simulink model "N3Z_tonetestprevious"  (R2014b)
settings: Solver=ode3  SolverMode=SingleTasking  StartTime=0.0  StopTime=1e-4  FixedStep=fpgaclk  RelTol=1e-3
PreLoadFcn:
  | %fpgaclk=1/32.768e6
  | fpgaclk=1/49.162e6
  | 
  | SerialData=[1,zeros(1,11),1,0,0,1]
  | load ../N3workingG/window
  | win=win';  %Go back to using flatter and wider windowed sync function
  | %load ../N3workingG/hanning    %use Hahn window
  | 
  | load ../N3workingG/PREemphasis   %For pre-empasis and deemphasis FIRs
  | 
  | %LUT3=xls2LUT2('../IQI_Qdemod.xls'); LUT3
  | load ../N3workingG/LUT3
  | load ../N3workingG/FIRiq2
  | % xls2LUT
  | 
  | GetProgFiles
  | 
  | PinAssignments    %Get Pin references for TE0722
  | 
  | 
  | 
  | 
  | 
  | %LCD
  | LCDdata=[LCD_D7,LCD_D6,LCD_D5,LCD_D4,LCD_D3,LCD_D2,LCD_D1,LCD_D0] %Note MSB...LSB!
  | LCDctrl=[LCD_E,LCD_RW,LCD_RS];
  | 
  | %for RS232 on pins 3 and 5 of USBB
  | 
  | %BT chip connections for WT12
  | 
  | RX_BT=RXD
  | TX_BT=TXD
  | 
  | RST_BB=RES
  | 
  | %PCMC=PCMC
  | %PCMS=PCMS
  | %PCMI=PCMI
  | %PCMO=PCMO
  | 
  | %Aliases:
  | SRDBT=PCMI
  | STDBT=PCMO
  | SCLK_BT=PCMC
  | SFS_BT=PCMS
  | 
  | %ADC control
  | 
  | %SDOA=SDOA
  | %SDOB=SDOB
  | %SCK=SCK
  | CONV=Csbar
  | CAL=Cal
  | 
  | ADC_G=[ADC_G3,ADC_G2,ADC_G1,ADC_G0]
  | %PD settings hard coded now
  | 
  | %%%%%%
  | TX_LOW=TX_Low
  | 
  | %Leds
  | %Defined inPinassignments
  | 
  | 
  | 
  | %TouchPads
  | %Defined in Pinassignments
  | load Snip16bSigned
  | 
  | 'Got to end of pre-load OK'
StartFcn:
  | SerialData=[1,zeros(1,11),1,0,0,1]
values from neighbouring files (symbols this model uses):
  ADC_G0 = {'P10'}    [PinAssignments.m]
  ADC_G1 = {'P11'}    [PinAssignments.m]
  ADC_G2 = {'N14'}    [PinAssignments.m]
  ADC_G3 = {'M11'}    [PinAssignments.m]
  Cal = {'L12'}    [PinAssignments.m]
  Csbar = {'M12'}    [PinAssignments.m]
  LCD_D0 = {'J13'}    [PinAssignments.m]
  LCD_D1 = {'J14'}    [PinAssignments.m]
  LCD_D2 = {'F15'}    [PinAssignments.m]
  LCD_D3 = {'H14'}    [PinAssignments.m]
  LCD_D4 = {'G12'}    [PinAssignments.m]
  LCD_D5 = {'L15'}    [PinAssignments.m]
  LCD_D6 = {'M14'}    [PinAssignments.m]
  LCD_D7 = {'K15'}    [PinAssignments.m]
  PCMC = {'H11'}    [PinAssignments.m]
  PCMI = {'H12'}    [PinAssignments.m]
  PCMO = {'N13'}    [PinAssignments.m]
  PCMS = {'M10'}    [PinAssignments.m]
  RES = {'G11'}    [PinAssignments.m]
  RXD = {'H13'}    [PinAssignments.m]
  TX_Low = {'P15'}    [PinAssignments.m]
  TXD = {'P13'}    [PinAssignments.m]
undefined symbols (not defined in the file or in its folder): AXI4, FIRRX, FIRTX, Lite
libraries: xbsIndex_r4 x1250, MyFunctions x43
(part 1 of 10)
settings Model: Creator=Graham  LastModifiedBy=gnaylor
settings DataIOCC: SignalLoggingName=sigsOut
settings OptimizationCC: ExpressionDepthLimit=2147483647  InitFltsAndDblsToZero=on
settings DebuggingCC: SaveWithParameterizedLinksMsg=none  UnderspecifiedInitializationDetection=Classic  MergeDetectMultiDrivingBlocksExec=none  SignalResolutionControl=TryResolveAllWithWarning  SolverPrmCheckMsg=none  MultiTaskDSMMsg=warning  MultiTaskCondExecSysMsg=none  FrameProcessingCompatibilityMsg=error  StateNameClashWarn=warning
settings HardwareCC: TargetUnknown=on
settings GRTTargetCC: TargetFcnLib=ansi_tfl_tmw.mat  ModelReferenceCompliant=off  CombineOutputUpdateFcns=off  MatFileLogging=off  GRTInterface=on

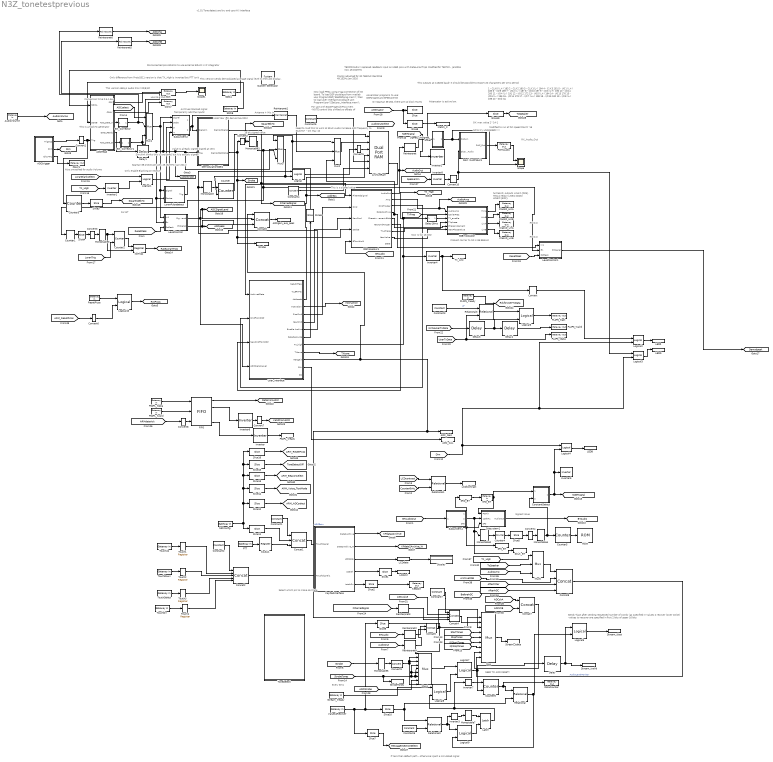
== system N3Z_tonetestprevious ==
  note: If zero then default path - otherwise inject a simulated signal
  note: Every 8ms
  note: Disconnected pico BRAMs to use external BRAM in IP integrator
  note: NEED TO ADD RESET!!
  note: Sends Tlast after sending requested number of words (as specified in Values 2 recover lower 16 bit)
      | -values to recover are specified in first 2 bits of upper 16 bits
  note: Also smoothed for audio Volume
  note: Modified to run at full speed March '16
  note: v1.01 Tone detect and try and use AXI interface
  note: OK max value 2^14-1
  note: This outputs at 115200 baud! It should be possible to export 20 characters per 2ms period
  note: 1 - CLK0 (L+)	183	2 - CLK2	180
      | 3 - CLK1(L-)	184	4 - CLK3	181
      | 5 - I/O1 (L+)	185	6 - I/O9	189
      | 7 - I/O2 (L-)	187	8 - I/O10	197
      | 9 - I/O3 (L+)	190	10 - I/O11	200
      | 11 - I/O4 (L-)	191	12 - I/O12	172
      | 13 - I/O5 (L+)	194	14 - I/O13	176
      | 15 - I/O6 (L-)	196	16 - I/O14	178
      | 17 - I/O7 (L+)	198	18 - I/O15	182
      | 19 - I/O8 (L-)	199	20 - Gnd	NA
  note: This is a 512kHz generator
  note: use 24.6 MHz
  note: Spartan 3E prototype uses 49.152MHz (Jan 2011)
  note: Conversion time 0.5-1.6us
  note: RX_Audio_Out
  note: RF Out
  note: Antenna + Mic In
  note: Now load FPGA using J-tag connection
      | of N3 board.
      | To load DSP picoblaze from matlab use:
      | ProgramDSP('S3eDSPprog.mem');
      | then to load user interface picoblaze use:
      | ProgramUser('S3eUser_interface.mem');
  note: Assembler programs to use:
      | DSPprogN3 and
      | SP3eUserN3
  note: Value is already signed biased at zero
  note: This is a signed value
  note: For use with BootProgMultiPico.mem
      | -NOTE control bits shifted so offsets of
  note: Need to mod this to work at 8kHz Audio
      | Increase ADC frequency to 512kHz? - OK May 10
  note: Closest carrier to N2 is 86.956kHz
  note: 18 bit signed value
  note: Simulink thinks this is unsigned, but it is actualy signed
  note: Clocks adjusted for 32.768MHz Dec2015
      | 49.152Mz Jan 2016
  note: Select which pin to make oscillate
  note: %ClassD_outputs
      | LINA={D25}
      | HINA={B24}
      | LINB={D23}
      | HINB={B22}
  note: RF Out
  note: On Spartan 3E 250, there are 12 block RAMs
  note: NOW try UNSIGNED!!!!!
  note: Temporarily add the inputs!
  note: Now is
      | full 16 bits!
  note: Only difference from Proto2011 version is that TX_High is inverted but PTT isn't
  note: Archives blanked signal
  note: Only enable Blanking on receive
  note: This version delays audio 2ms (20/8/12)
  note: Uses new I_Q demod Nov2012
  note: TEMPORARILY replaced readback input on USER pico with RateLoranTrips
      | Modified for TE0722 - Jan2016 now 49.152MHz
  note: Signed Value
  note: For BT
  note: Attenuator is active low.
  note: This version sends demodulated average signal level to the LCD display.
  " System Generator" : xbsIndex_r4/ System Generator  Tag=genX  xilinxfamily=zynq  part=xc7z010  speed=-1  package=clg225  synthesis_tool=XST  clock_wrapper=Clock Enables  directory=../SysgenOutput/TE0722/ToneDetect2  proj_type=Project Navigator  Synth_file=XST Defaults  Impl_file=ISE Defaults  testbench=off  simulink_period=fpgaclk  sysclk_period=1e9*fpgaclk  dcm_input_clock_period=100  incr_netlist=off  trim_vbits=Everywhere in SubSystem  dbl_ovrd=According to Block Masks  core_generation=According to Block Masks  run_coregen=off  deprecated_control=off  eval_field=0  block_type=sysgen
      settings: block_version=8.2.02
  ADCRead : Subsystem
  ADC_CAL : xbsIndex_r4/Gateway Out  inherit_from_input=off  hdl_port=on  rows=1  columns=1  UseAsDAC=off  DACChannel='1'  interface=None  automatic_assignment=on  address_offset=hex2dec('00')  intf_name=''  intf_description=''  timing_constraint=None  locs_specified=off  LOCs=CAL  io_standard={'LVCMOS33'}  block_type=gatewayout
      settings: block_version=VER_STRING_GOES_HERE
  ADC_Gain : xbsIndex_r4/Gateway Out  inherit_from_input=off  hdl_port=on  rows=1  columns=1  UseAsDAC=off  DACChannel='1'  interface=None  automatic_assignment=on  address_offset=hex2dec('00')  intf_name=''  intf_description=''  timing_constraint=None  locs_specified=on  LOCs=ADC_G  io_standard={'LVCMOS','LVCMOS','LVCMOS','LVCMOS'}  block_type=gatewayout
      settings: block_version=VER_STRING_GOES_HERE
  ADCgain_ave_peak : xbsIndex_r4/Gateway Out  inherit_from_input=off  hdl_port=on  rows=1  columns=1  UseAsDAC=off  DACChannel='1'  interface=AXI4-Lite  automatic_assignment=on  address_offset=hex2dec('00')  intf_name=''  intf_description=''  timing_constraint=None  locs_specified=on  LOCs=Strobe  io_standard={'LVCMOS33'}  block_type=gatewayout
      settings: block_version=VER_STRING_GOES_HERE
  ADCtrigger : Subsystem
  ArchiveRam : xbsIndex_r4/Dual Port RAM  depth=1024*2  initVector=zeros(1,4096)  distributed_mem=Block RAM  init_a=0  init_b=0  rst_a=off  rst_b=off  en_a=off  en_b=off  latency=1  write_mode_A=Read After Write  write_mode_B=Read After Write  optimize=Area  dbl_ovrd=off  block_type=dpram
      settings: block_version=8.2.02
  AudioVolume : xbsIndex_r4/Gateway In  gui_display_data_type=Fixed-point  arith_type=Unsigned  n_bits=9  bin_pt=0  preci_type=Single  exp_width=8  frac_width=24  rows=1  columns=1  quantization="Round  (unbiased: +/- Inf)"  overflow=Saturate  period=fpgaclk  UseAsADC=off  ADCChannel='1'  interface=AXI4-Lite  automatic_assignment=on  address_offset=hex2dec('00')  intf_name=''  intf_description=''  default_value=0  timing_constraint=None  locs_specified=off  LOCs=RS232rx  io_standard={'LVCMOS33'}  inherit_from_input=off  hdl_port=on  dbl_ovrd=off  block_type=gatewayin
      settings: block_version=VER_STRING_GOES_HERE
  Bit_Corrector : Subsystem  TreatAsAtomicUnit=on
  Bit_Corrector1 : Subsystem  TreatAsAtomicUnit=on
  CONV : xbsIndex_r4/Gateway Out  inherit_from_input=off  hdl_port=on  rows=1  columns=1  UseAsDAC=off  DACChannel='1'  interface=None  automatic_assignment=on  address_offset=hex2dec('00')  intf_name=''  intf_description=''  timing_constraint=None  locs_specified=on  LOCs=CONV  io_standard={'LVCMOS33'}  block_type=gatewayout
      settings: xl_area=[0, 0, 0, 0, 0, 0, 0]  block_version=VER_STRING_GOES_HERE
  ClassD_HinA : xbsIndex_r4/Gateway Out  inherit_from_input=off  hdl_port=on  rows=1  columns=1  UseAsDAC=off  DACChannel='1'  interface=None  automatic_assignment=on  address_offset=hex2dec('00')  intf_name=''  intf_description=''  timing_constraint=None  locs_specified=on  LOCs=HINA  io_standard={'LVCMOS33'}  block_type=gatewayout
      settings: xl_area=[0, 0, 0, 0, 0, 0, 0]  block_version=VER_STRING_GOES_HERE
  ClassD_HinB : xbsIndex_r4/Gateway Out  inherit_from_input=off  hdl_port=on  rows=1  columns=1  UseAsDAC=off  DACChannel='1'  interface=None  automatic_assignment=on  address_offset=hex2dec('00')  intf_name=''  intf_description=''  timing_constraint=None  locs_specified=on  LOCs=HINB  io_standard={'LVCMOS33'}  block_type=gatewayout
      settings: xl_area=[0, 0, 0, 0, 0, 0, 0]  block_version=VER_STRING_GOES_HERE
  ClassD_LinA : xbsIndex_r4/Gateway Out  inherit_from_input=off  hdl_port=on  rows=1  columns=1  UseAsDAC=off  DACChannel='1'  interface=None  automatic_assignment=on  address_offset=hex2dec('00')  intf_name=''  intf_description=''  timing_constraint=None  locs_specified=on  LOCs=LINA  io_standard={'LVCMOS33'}  block_type=gatewayout
      settings: xl_area=[0, 0, 0, 0, 0, 0, 0]  block_version=VER_STRING_GOES_HERE
  ClassD_LinB : xbsIndex_r4/Gateway Out  inherit_from_input=off  hdl_port=on  rows=1  columns=1  UseAsDAC=off  DACChannel='1'  interface=None  automatic_assignment=on  address_offset=hex2dec('00')  intf_name=''  intf_description=''  timing_constraint=None  locs_specified=on  LOCs=LINB  io_standard={'LVCMOS33'}  block_type=gatewayout
      settings: xl_area=[0, 0, 0, 0, 0, 0, 0]  block_version=VER_STRING_GOES_HERE
  Concat1 : xbsIndex_r4/Concat  num_inputs=3  dbl_ovrd=off  block_type=concat
      settings: block_version=12.2
  Concat2 : xbsIndex_r4/Concat  num_inputs=5  dbl_ovrd=off  block_type=concat
      settings: block_version=12.2
  Concat4 : xbsIndex_r4/Concat  num_inputs=4  dbl_ovrd=off  block_type=concat
  Concat5 : xbsIndex_r4/Concat  num_inputs=2  dbl_ovrd=off  block_type=concat
  Concat6 : xbsIndex_r4/Concat  num_inputs=3  dbl_ovrd=off  block_type=concat
  Concat7 : xbsIndex_r4/Concat  num_inputs=2  dbl_ovrd=off  block_type=concat
  Concat8 : xbsIndex_r4/Concat  num_inputs=4  dbl_ovrd=off  block_type=concat
  Constant1 : xbsIndex_r4/Constant  const=0  gui_display_data_type=Fixed-point  arith_type=Unsigned  n_bits=4  bin_pt=0  preci_type=Single  exp_width=8  frac_width=24  explicit_period=on  period=fpgaclk  equ=P=C  opselect=C  inp2=PCIN>>17  opr=+  inp1=P  carry=CIN  dbl_ovrd=off  block_type=constant
      settings: block_version=VER_STRING_GOES_HERE
  Constant2 : xbsIndex_r4/Constant  const=0  gui_display_data_type=Fixed-point  arith_type=Unsigned  n_bits=4  bin_pt=0  preci_type=Single  exp_width=8  frac_width=24  explicit_period=on  period=fpgaclk  equ=P=C  opselect=C  inp2=PCIN>>17  opr=+  inp1=P  carry=CIN  dbl_ovrd=off  block_type=constant
      settings: block_version=VER_STRING_GOES_HERE
  Constant3 : xbsIndex_r4/Constant  const=10  gui_display_data_type=Fixed-point  arith_type=Unsigned  n_bits=8  bin_pt=0  preci_type=Single  exp_width=8  frac_width=24  explicit_period=off  period=1  equ=P=C  opselect=C  inp2=PCIN>>17  opr=+  inp1=P  carry=CIN  dbl_ovrd=off  block_type=constant
  Constant4 : xbsIndex_r4/Constant  const=0  gui_display_data_type=Boolean  arith_type=Boolean  n_bits=1  bin_pt=0  preci_type=Single  exp_width=8  frac_width=24  explicit_period=on  period=fpgaclk  equ=P=C  opselect=C  inp2=PCIN>>17  opr=+  inp1=P  carry=CIN  dbl_ovrd=off  block_type=constant
      settings: block_version=VER_STRING_GOES_HERE
  Constant5 : xbsIndex_r4/Constant  const=0  gui_display_data_type=Fixed-point  arith_type=Unsigned  n_bits=16  bin_pt=0  preci_type=Single  exp_width=8  frac_width=24  explicit_period=on  period=fpgaclk  equ=P=C  opselect=C  inp2=PCIN>>17  opr=+  inp1=P  carry=CIN  dbl_ovrd=off  block_type=constant
      settings: block_version=VER_STRING_GOES_HERE
  Constant6 : xbsIndex_r4/Constant  const=0  gui_display_data_type=Fixed-point  arith_type=Unsigned  n_bits=16  bin_pt=0  preci_type=Single  exp_width=8  frac_width=24  explicit_period=on  period=fpgaclk  equ=P=C  opselect=C  inp2=PCIN>>17  opr=+  inp1=P  carry=CIN  dbl_ovrd=off  block_type=constant
  Constant7 : xbsIndex_r4/Constant  const=0  gui_display_data_type=Fixed-point  arith_type=Unsigned  n_bits=2  bin_pt=0  preci_type=Single  exp_width=8  frac_width=24  explicit_period=on  period=fpgaclk  equ=P=C  opselect=C  inp2=PCIN>>17  opr=+  inp1=P  carry=CIN  dbl_ovrd=off  block_type=constant
  ConstantDetect : Subsystem
  Convert : xbsIndex_r4/Convert  gui_display_data_type=Boolean  arith_type=Boolean  n_bits=16  bin_pt=14  float_type=Single  exp_bits=8  fraction_bits=24  quantization=Truncate  overflow=Wrap  en=off  latency=0  pipeline=off  dbl_ovrd=off  block_type=convert
      settings: block_version=8.2.02
  Convert1 : xbsIndex_r4/Convert  gui_display_data_type=Boolean  arith_type=Boolean  n_bits=8  bin_pt=6  float_type=Single  exp_bits=8  fraction_bits=24  quantization=Truncate  overflow=Wrap  en=off  latency=0  pipeline=off  dbl_ovrd=off  block_type=convert
      settings: xl_area=[0 0 0 0 0 0 0]  block_version=VER_STRING_GOES_HERE
  Convert10 : xbsIndex_r4/Convert  gui_display_data_type=Boolean  arith_type=Boolean  n_bits=16  bin_pt=14  float_type=Single  exp_bits=8  fraction_bits=24  quantization=Truncate  overflow=Wrap  en=off  latency=0  pipeline=off  dbl_ovrd=off  block_type=convert
      settings: block_version=8.2.02
  Convert2 : xbsIndex_r4/Convert  gui_display_data_type=Boolean  arith_type=Boolean  n_bits=16  bin_pt=0  float_type=Single  exp_bits=8  fraction_bits=24  quantization=Truncate  overflow=Wrap  en=off  latency=0  pipeline=off  dbl_ovrd=off  block_type=convert
      settings: xl_area=[0, 0, 0, 0, 0, 0, 0]  block_version=VER_STRING_GOES_HERE
  Convert3 : xbsIndex_r4/Convert  gui_display_data_type=Fixed-point  arith_type=Boolean  n_bits=16  bin_pt=14  float_type=Single  exp_bits=8  fraction_bits=24  quantization=Truncate  overflow=Wrap  en=off  latency=0  pipeline=off  dbl_ovrd=off  block_type=convert
      settings: block_version=8.2.02
  Convert4 : xbsIndex_r4/Convert  gui_display_data_type=Fixed-point  arith_type=Boolean  n_bits=8  bin_pt=6  float_type=Single  exp_bits=8  fraction_bits=24  quantization=Truncate  overflow=Wrap  en=off  latency=0  pipeline=off  dbl_ovrd=off  block_type=convert
      settings: xl_area=[0 0 0 0 0 0 0]  block_version=VER_STRING_GOES_HERE
  Convert5 : xbsIndex_r4/Convert  gui_display_data_type=Fixed-point  arith_type=Boolean  n_bits=16  bin_pt=14  float_type=Single  exp_bits=8  fraction_bits=24  quantization=Truncate  overflow=Wrap  en=off  latency=0  pipeline=off  dbl_ovrd=off  block_type=convert
      settings: block_version=8.2.02
  Convert6 : xbsIndex_r4/Convert  gui_display_data_type=Boolean  arith_type=Boolean  n_bits=8  bin_pt=6  float_type=Single  exp_bits=8  fraction_bits=24  quantization=Truncate  overflow=Wrap  en=off  latency=0  pipeline=off  dbl_ovrd=off  block_type=convert
      settings: xl_area=[0 0 0 0 0 0 0]  block_version=VER_STRING_GOES_HERE
  Convert7 : xbsIndex_r4/Convert  gui_display_data_type=Fixed-point  arith_type=Unsigned  n_bits=1  bin_pt=0  float_type=Single  exp_bits=8  fraction_bits=24  quantization=Truncate  overflow=Wrap  en=off  latency=0  pipeline=off  dbl_ovrd=off  block_type=convert
      settings: block_version=8.2.02
  Convert8 : xbsIndex_r4/Convert  gui_display_data_type=Boolean  arith_type=Boolean  n_bits=1  bin_pt=0  float_type=Single  exp_bits=8  fraction_bits=24  quantization=Truncate  overflow=Wrap  en=off  latency=0  pipeline=off  dbl_ovrd=off  block_type=convert
      settings: block_version=8.2.02
  Convert9 : xbsIndex_r4/Convert  gui_display_data_type=Boolean  arith_type=Boolean  n_bits=16  bin_pt=14  float_type=Single  exp_bits=8  fraction_bits=24  quantization=Truncate  overflow=Wrap  en=off  latency=1  pipeline=off  dbl_ovrd=off  block_type=convert
  Counter : xbsIndex_r4/Counter  cnt_type=Free Running  cnt_to=Inf  operation=Up  start_count=0  cnt_by_val=1  arith_type=Unsigned  n_bits=11  bin_pt=0  load_pin=off  rst=on  en=on  explicit_period=off  period=1  use_behavioral_HDL=off  implementation=Fabric  use_rpm=off  dbl_ovrd=off  block_type=counter
      settings: block_version=8.2.02
  Counter1 : xbsIndex_r4/Counter  cnt_type=Free Running  cnt_to=Inf  operation=Up  start_count=0  cnt_by_val=1  arith_type=Unsigned  n_bits=13  bin_pt=0  load_pin=off  rst=off  en=on  explicit_period=off  period=1  use_behavioral_HDL=off  implementation=Fabric  use_rpm=off  dbl_ovrd=off  block_type=counter
      settings: block_version=8.2.02
  Counter2 : xbsIndex_r4/Counter  cnt_type=Free Running  cnt_to=Inf  operation=Up  start_count=0  cnt_by_val=1  arith_type=Unsigned  n_bits=8  bin_pt=0  load_pin=off  rst=on  en=on  explicit_period=off  period=1  use_behavioral_HDL=off  implementation=Fabric  use_rpm=off  dbl_ovrd=off  block_type=counter
      settings: block_version=8.2.02
  Counter3 : xbsIndex_r4/Counter  cnt_type=Free Running  cnt_to=Inf  operation=Up  start_count=0  cnt_by_val=1  arith_type=Unsigned  n_bits=2  bin_pt=0  load_pin=off  rst=off  en=on  explicit_period=on  period=fpgaclk  use_behavioral_HDL=off  implementation=Fabric  dbl_ovrd=off  block_type=counter
      settings: block_version=12.2
  Counter4 : xbsIndex_r4/Counter  cnt_type=Free Running  cnt_to=Inf  operation=Up  start_count=0  cnt_by_val=1  arith_type=Unsigned  n_bits=4  bin_pt=0  load_pin=off  rst=off  en=on  explicit_period=on  period=fpgaclk  use_behavioral_HDL=off  implementation=Fabric  dbl_ovrd=off  block_type=counter
      settings: block_version=12.2
  Counter5 : xbsIndex_r4/Counter  cnt_type=Free Running  cnt_to=Inf  operation=Up  start_count=0  cnt_by_val=1  arith_type=Unsigned  n_bits=4  bin_pt=0  load_pin=off  rst=off  en=on  explicit_period=on  period=fpgaclk  use_behavioral_HDL=off  implementation=Fabric  dbl_ovrd=off  block_type=counter
  Counter6 : xbsIndex_r4/Counter  cnt_type=Free Running  cnt_to=Inf  operation=Up  start_count=0  cnt_by_val=1  arith_type=Unsigned  n_bits=16  bin_pt=0  load_pin=off  rst=on  en=on  explicit_period=on  period=fpgaclk  use_behavioral_HDL=off  implementation=Fabric  dbl_ovrd=off  block_type=counter
  CoutA1 : xbsIndex_r4/Register  init=0  rst=off  en=off  dbl_ovrd=off  block_type=register
      settings: xl_area=[0, 0, 0, 0, 0, 0, 0]  block_version=VER_STRING_GOES_HERE
  DAC (XAPP154)1 : Subsystem
  DSProcessor1 : Subsystem
  DataCounter : xbsIndex_r4/Gateway Out  inherit_from_input=off  hdl_port=on  rows=1  columns=1  UseAsDAC=off  DACChannel='1'  interface=None  automatic_assignment=on  address_offset=hex2dec('00')  intf_name=''  intf_description=''  timing_constraint=None  locs_specified=off  LOCs=Keep_On  io_standard={'LVCMOS33'}  block_type=gatewayout
      settings: xl_area=[0, 0, 0, 0, 0, 0, 0]  block_version=VER_STRING_GOES_HERE
  Delay : xbsIndex_r4/Delay  rst=off  infoeditControl=Selection of Reset will increase slice count due to use of real FFs and instead of SRLs  en=off  latency=2  reg_retiming=off  dbl_ovrd=off  block_type=delay
      settings: infoedit=Hardware notes: A delay line is a chain, each link of which is an SRL16 or SRL32 followed by a flip-flop.
  Delay1 : xbsIndex_r4/Delay  rst=off  infoeditControl=Selection of Reset will increase slice count due to use of real FFs and instead of SRLs  en=off  latency=2  reg_retiming=off  dbl_ovrd=off  block_type=delay
      settings: xl_area=[1 1 0 0 0 0 0]  block_version=VER_STRING_GOES_HERE
  Delay16ms : Subsystem
  Delay3 : xbsIndex_r4/Delay  rst=off  infoeditControl=Selection of Reset will increase slice count due to use of real FFs and instead of SRLs  en=off  latency=2  reg_retiming=off  dbl_ovrd=off  block_type=delay
      settings: infoedit=Hardware notes: A delay line is a chain, each link of which is an SRL16 or SRL32 followed by a flip-flop.
  Delay4 : xbsIndex_r4/Delay  rst=off  infoeditControl=Selection of Reset will increase slice count due to use of real FFs and instead of SRLs  en=off  latency=1  reg_retiming=off  dbl_ovrd=off  block_type=delay
      settings: infoedit=Hardware notes: A delay line is a chain, each link of which is an SRL16 or SRL32 followed by a flip-flop.
  DemodulationSSB1 : Subsystem
  Display : Display
  FIFO : xbsIndex_r4/FIFO  mem_type=Block RAM  performance_options=First_Word_Fall_Through  embedded_registers=on  depth=16  percent_nbits=1  rst=off  rst_latency=1  en=off  use_dcount=off  use_percent_full_port=off  use_almost_empty=off  almost_empty_thresh=2  use_almost_full=on  almost_full_thresh=14  explicit_period=off  dbl_ovrd=off  block_type=fifo
  Inverter{,1..2,4..6,8} (7 alike) : xbsIndex_r4/Inverter  en=off  latency=0  dbl_ovrd=off  block_type=inv
      Inverter1 settings: block_version=12.2
      Inverter2 settings: block_version=12.2
      Inverter4 settings: block_version=12.2
      Inverter5 settings: block_version=12.2
      Inverter8 settings: block_version=12.2
  Inverter3 : xbsIndex_r4/Inverter  en=off  latency=1  dbl_ovrd=off  block_type=inv
  Inverter7 : xbsIndex_r4/Inverter  en=off  latency=1  dbl_ovrd=off  block_type=inv
  KeepOn : xbsIndex_r4/Gateway Out  inherit_from_input=off  hdl_port=on  rows=1  columns=1  UseAsDAC=off  DACChannel='1'  interface=None  automatic_assignment=on  address_offset=hex2dec('00')  intf_name=''  intf_description=''  timing_constraint=None  locs_specified=on  LOCs=Keep_On  io_standard={'LVCMOS33'}  block_type=gatewayout
      settings: xl_area=[0, 0, 0, 0, 0, 0, 0]  block_version=VER_STRING_GOES_HERE
  KeyPadinterface : Subsystem
  LCDContrast : xbsIndex_r4/Gateway Out  inherit_from_input=off  hdl_port=on  rows=1  columns=1  UseAsDAC=off  DACChannel='1'  interface=None  automatic_assignment=on  address_offset=hex2dec('00')  intf_name=''  intf_description=''  timing_constraint=None  locs_specified=on  LOCs=LCD_V0  io_standard={'LVCMOS33'}  block_type=gatewayout
      settings: block_version=VER_STRING_GOES_HERE
  LCDctrl : xbsIndex_r4/Gateway Out  inherit_from_input=off  hdl_port=on  rows=1  columns=1  UseAsDAC=off  DACChannel='1'  interface=None  automatic_assignment=on  address_offset=hex2dec('00')  intf_name=''  intf_description=''  timing_constraint=None  locs_specified=on  LOCs=LCDctrl  io_standard={'LVCMOS33','LVCMOS33','LVCMOS33'}  block_type=gatewayout
      settings: block_version=VER_STRING_GOES_HERE
  LCDdata : xbsIndex_r4/Gateway Out  inherit_from_input=off  hdl_port=on  rows=1  columns=1  UseAsDAC=off  DACChannel='1'  interface=None  automatic_assignment=on  address_offset=hex2dec('00')  intf_name=''  intf_description=''  timing_constraint=None  locs_specified=on  LOCs=LCDdata  io_standard={'LVCMOS33','LVCMOS33','LVCMOS33','LVCMOS33','LVCMOS33','LVCMOS33','LVCMOS33','LVCMOS33'}  block_type=gatewayout
      settings: block_version=VER_STRING_GOES_HERE
  LEDB : xbsIndex_r4/Gateway Out  inherit_from_input=off  hdl_port=on  rows=1  columns=1  UseAsDAC=off  DACChannel='1'  interface=None  automatic_assignment=on  address_offset=hex2dec('00')  intf_name=''  intf_description=''  timing_constraint=None  locs_specified=on  LOCs=RGB_B  io_standard={'LVCMOS33'}  block_type=gatewayout
      settings: block_version=VER_STRING_GOES_HERE
  LEDG : xbsIndex_r4/Gateway Out  inherit_from_input=off  hdl_port=on  rows=1  columns=1  UseAsDAC=off  DACChannel='1'  interface=None  automatic_assignment=on  address_offset=hex2dec('00')  intf_name=''  intf_description=''  timing_constraint=None  locs_specified=on  LOCs=RGB_G  io_standard={'LVCMOS33'}  block_type=gatewayout
      settings: block_version=VER_STRING_GOES_HERE
  LEDR : xbsIndex_r4/Gateway Out  inherit_from_input=off  hdl_port=on  rows=1  columns=1  UseAsDAC=off  DACChannel='1'  interface=None  automatic_assignment=on  address_offset=hex2dec('00')  intf_name=''  intf_description=''  timing_constraint=None  locs_specified=on  LOCs=RGB_R  io_standard={'LVCMOS33'}  block_type=gatewayout
      settings: block_version=VER_STRING_GOES_HERE
  Latch : MyFunctions/Latch
  LevelMonitor : Subsystem
  LevelMonitor1 : Subsystem
  Logical : xbsIndex_r4/Logical  logical_function=AND  inputs=2  en=off  latency=2  precision=Full  arith_type=Unsigned  n_bits=16  bin_pt=0  align_bp=on  dbl_ovrd=off  block_type=logical
      settings: block_version=8.2.02
  Logical1 : xbsIndex_r4/Logical  logical_function=AND  inputs=2  en=off  latency=1  precision=Full  arith_type=Unsigned  n_bits=16  bin_pt=0  align_bp=on  dbl_ovrd=off  block_type=logical
      settings: block_version=8.2.02
  Logical{2..4,10} (4 alike) : xbsIndex_r4/Logical  logical_function=OR  inputs=2  en=off  latency=1  precision=Full  arith_type=Unsigned  n_bits=16  bin_pt=0  align_bp=on  dbl_ovrd=off  block_type=logical
  Logical5 : xbsIndex_r4/Logical  logical_function=AND  inputs=2  en=off  latency=0  precision=Full  arith_type=Unsigned  n_bits=16  bin_pt=0  align_bp=on  dbl_ovrd=off  block_type=logical
  Logical6 : xbsIndex_r4/Logical  logical_function=AND  inputs=2  en=off  latency=1  precision=Full  arith_type=Unsigned  n_bits=16  bin_pt=0  align_bp=on  dbl_ovrd=off  block_type=logical
  Logical7 : xbsIndex_r4/Logical  logical_function=AND  inputs=2  en=off  latency=1  precision=Full  arith_type=Unsigned  n_bits=16  bin_pt=0  align_bp=on  dbl_ovrd=off  block_type=logical
  Logical8 : xbsIndex_r4/Logical  logical_function=AND  inputs=2  en=off  latency=0  precision=Full  arith_type=Unsigned  n_bits=16  bin_pt=0  align_bp=on  dbl_ovrd=off  block_type=logical
  Logical9 : xbsIndex_r4/Logical  logical_function=OR  inputs=2  en=off  latency=0  precision=Full  arith_type=Unsigned  n_bits=16  bin_pt=0  align_bp=on  dbl_ovrd=off  block_type=logical
  LoranPulsedetect : Subsystem
  Match_Z : xbsIndex_r4/Gateway Out  inherit_from_input=off  hdl_port=on  rows=1  columns=1  UseAsDAC=off  DACChannel='1'  interface=None  automatic_assignment=on  address_offset=hex2dec('00')  intf_name=''  intf_description=''  timing_constraint=None  locs_specified=on  LOCs=MatchZ  io_standard={'LVCMOS33'}  block_type=gatewayout
      settings: block_version=VER_STRING_GOES_HERE
  Monostable : MyFunctions/Monostable
  Monostable1 : MyFunctions/Monostable
      link override Delay1: en=off  latency=1  dbl_ovrd=off  reg_retiming=off
      link override Delay1: infoedit=Hardware notes: A delay line is a chain, each link of which is an SRL16 followed by a flip-flop.  xl_area=[0, 0, 0, 0, 0, 0, 0]
  Monostable2 : MyFunctions/Monostable
      link override Delay1: xl_area=[1 1 0 0 0 0 0]
      link override Inverter: xl_area=[0 0 0 0 0 0 0]
      link override Logical: xl_area=[1 0 0 1 0 0 0]
  Monostable3 : MyFunctions/Monostable
      link override Delay1: en=off  latency=1  dbl_ovrd=off  reg_retiming=off
      link override Delay1: infoedit=Hardware notes: A delay line is a chain, each link of which is an SRL16 followed by a flip-flop.  xl_area=[0, 0, 0, 0, 0, 0, 0]
  Monostable4 : MyFunctions/Monostable
      link override Delay1: xl_area=[1 1 0 0 0 0 0]
      link override Inverter: xl_area=[0 0 0 0 0 0 0]
      link override Logical: xl_area=[1 0 0 1 0 0 0]
  Monostable5 : MyFunctions/Monostable
      link override Delay1: en=off  latency=1  dbl_ovrd=off  reg_retiming=off
      link override Delay1: infoedit=Hardware notes: A delay line is a chain, each link of which is an SRL16 followed by a flip-flop.  xl_area=[0, 0, 0, 0, 0, 0, 0]
  Monostable7 : MyFunctions/Monostable
      link override Delay1: en=off  latency=1  dbl_ovrd=off  reg_retiming=off
      link override Delay1: infoedit=Hardware notes: A delay line is a chain, each link of which is an SRL16 followed by a flip-flop.  xl_area=[0, 0, 0, 0, 0, 0, 0]
  Mux : xbsIndex_r4/Mux  inputs=8  en=off  latency=1  precision=Full  arith_type=Unsigned  n_bits=16  bin_pt=14  quantization=Truncate  overflow=Wrap  dbl_ovrd=off  block_type=mux
  Mux{1..3,5} (4 alike) : xbsIndex_r4/Mux  inputs=2  en=off  latency=1  precision=Full  arith_type=Unsigned  n_bits=16  bin_pt=14  quantization=Truncate  overflow=Wrap  dbl_ovrd=off  block_type=mux
      Mux1 settings: block_version=VER_STRING_GOES_HERE
      Mux2 settings: block_version=VER_STRING_GOES_HERE
      Mux3 settings: block_version=VER_STRING_GOES_HERE
  Mux4 : xbsIndex_r4/Mux  inputs=8  en=off  latency=1  precision=Full  arith_type=Unsigned  n_bits=16  bin_pt=14  quantization=Truncate  overflow=Wrap  dbl_ovrd=off  block_type=mux
  N3Zconfig : xbsIndex_r4/Gateway In  gui_display_data_type=Fixed-point  arith_type=Unsigned  n_bits=32  bin_pt=0  preci_type=Single  exp_width=8  frac_width=24  rows=1  columns=1  quantization=Truncate  overflow=Saturate  period=fpgaclk  UseAsADC=off  ADCChannel='1'  interface=AXI4-Lite  automatic_assignment=on  address_offset=hex2dec('00')  intf_name=''  intf_description=''  default_value=0  timing_constraint=None  locs_specified=off  LOCs=PTT  io_standard={'LVCMOS33'}  inherit_from_input=off  hdl_port=on  dbl_ovrd=off  block_type=gatewayin
      settings: xl_area=[0, 0, 0, 0, 0, 0, 0]  block_version=VER_STRING_GOES_HERE
  NoTrips : xbsIndex_r4/Register  init=0  rst=off  en=on  dbl_ovrd=off  block_type=register
      settings: xl_area=[0, 0, 0, 0, 0, 0, 0]  block_version=VER_STRING_GOES_HERE
  PL2PS_tdata : xbsIndex_r4/Gateway Out  inherit_from_input=off  hdl_port=on  rows=1  columns=1  UseAsDAC=off  DACChannel='1'  interface=None  automatic_assignment=on  address_offset=hex2dec('00')  intf_name=''  intf_description=''  timing_constraint=None  locs_specified=off  LOCs={}  io_standard={}  block_type=gatewayout
  PL2PS_tlast : xbsIndex_r4/Gateway Out  inherit_from_input=off  hdl_port=on  rows=1  columns=1  UseAsDAC=off  DACChannel='1'  interface=None  automatic_assignment=on  address_offset=hex2dec('00')  intf_name=''  intf_description=''  timing_constraint=None  locs_specified=off  LOCs={}  io_standard={}  block_type=gatewayout
  PL2PS_tready : xbsIndex_r4/Gateway In  gui_display_data_type=Boolean  arith_type=Boolean  n_bits=1  bin_pt=0  preci_type=Single  exp_width=8  frac_width=24  rows=1  columns=1  quantization="Round  (unbiased: +/- Inf)"  overflow=Wrap  period=fpgaclk  UseAsADC=off  ADCChannel='1'  interface=None  automatic_assignment=on  address_offset=hex2dec('00')  intf_name=''  intf_description=''  default_value=0  timing_constraint=None  locs_specified=off  LOCs=RS232rx  io_standard={'LVCMOS33'}  inherit_from_input=off  hdl_port=on  dbl_ovrd=off  block_type=gatewayin
      settings: block_version=VER_STRING_GOES_HERE
  PL2PS_tvalid : xbsIndex_r4/Gateway Out  inherit_from_input=off  hdl_port=on  rows=1  columns=1  UseAsDAC=off  DACChannel='1'  interface=None  automatic_assignment=on  address_offset=hex2dec('00')  intf_name=''  intf_description=''  timing_constraint=None  locs_specified=off  LOCs={}  io_standard={}  block_type=gatewayout
  PS2PL_tdata : xbsIndex_r4/Gateway In  gui_display_data_type=Fixed-point  arith_type=Unsigned  n_bits=8  bin_pt=0  preci_type=Single  exp_width=8  frac_width=24  rows=1  columns=1  quantization="Round  (unbiased: +/- Inf)"  overflow=Wrap  period=fpgaclk  UseAsADC=off  ADCChannel='1'  interface=None  automatic_assignment=on  address_offset=hex2dec('00')  intf_name=''  intf_description=''  default_value=0  timing_constraint=None  locs_specified=off  LOCs=RS232rx  io_standard={'LVCMOS33'}  inherit_from_input=off  hdl_port=on  dbl_ovrd=off  block_type=gatewayin
      settings: block_version=VER_STRING_GOES_HERE
  PS2PL_tready : xbsIndex_r4/Gateway Out  inherit_from_input=off  hdl_port=on  rows=1  columns=1  UseAsDAC=off  DACChannel='1'  interface=None  automatic_assignment=on  address_offset=hex2dec('00')  intf_name=''  intf_description=''  timing_constraint=None  locs_specified=off  LOCs=RST_BB  io_standard={'LVCMOS'}  block_type=gatewayout
      settings: block_version=VER_STRING_GOES_HERE
  PS2PL_tvalid : xbsIndex_r4/Gateway In  gui_display_data_type=Boolean  arith_type=Boolean  n_bits=1  bin_pt=0  preci_type=Single  exp_width=8  frac_width=24  rows=1  columns=1  quantization="Round  (unbiased: +/- Inf)"  overflow=Wrap  period=fpgaclk  UseAsADC=off  ADCChannel='1'  interface=None  automatic_assignment=on  address_offset=hex2dec('00')  intf_name=''  intf_description=''  default_value=0  timing_constraint=None  locs_specified=off  LOCs=RS232rx  io_standard={'LVCMOS33'}  inherit_from_input=off  hdl_port=on  dbl_ovrd=off  block_type=gatewayin
      settings: block_version=VER_STRING_GOES_HERE
  PSUclk : xbsIndex_r4/Gateway Out  inherit_from_input=off  hdl_port=on  rows=1  columns=1  UseAsDAC=off  DACChannel='1'  interface=None  automatic_assignment=on  address_offset=hex2dec('00')  intf_name=''  intf_description=''  timing_constraint=None  locs_specified=off  LOCs={}  io_standard={}  block_type=gatewayout
  PTT : xbsIndex_r4/Gateway In  gui_display_data_type=Fixed-point  arith_type=Unsigned  n_bits=1  bin_pt=0  preci_type=Single  exp_width=8  frac_width=24  rows=1  columns=1  quantization=Truncate  overflow=Saturate  period=fpgaclk  UseAsADC=off  ADCChannel='1'  interface=None  automatic_assignment=on  address_offset=hex2dec('00')  intf_name=''  intf_description=''  default_value=0  timing_constraint=None  locs_specified=on  LOCs=PTT  io_standard={'LVCMOS33'}  inherit_from_input=off  hdl_port=on  dbl_ovrd=off  block_type=gatewayin
      settings: xl_area=[0, 0, 0, 0, 0, 0, 0]  block_version=VER_STRING_GOES_HERE
  PWMAudio : xbsIndex_r4/Gateway Out  inherit_from_input=off  hdl_port=on  rows=1  columns=1  UseAsDAC=off  DACChannel='1'  interface=None  automatic_assignment=on  address_offset=hex2dec('00')  intf_name=''  intf_description=''  timing_constraint=None  locs_specified=on  LOCs=PWMAudio  io_standard={'LVCMOS33'}  block_type=gatewayout
      settings: xl_area=[0, 0, 0, 0, 0, 0, 0]  block_version=VER_STRING_GOES_HERE
  ROM : xbsIndex_r4/ROM  depth=16  initVector=(2^14-2^12)*sin(pi*(0:15)/8)  distributed_mem=Distributed memory  rst=off  init_reg=0  en=off  latency=1  gui_display_data_type=Fixed-point  arith_type="Signed  (2's comp)"  n_bits=16  bin_pt=0  preci_type=Single  exp_width=8  frac_width=24  optimize=Area  use_rpm=on  dbl_ovrd=off  block_type=sprom
  Reinterpret : xbsIndex_r4/Reinterpret  force_arith_type=on  arith_type="Signed  (2's comp)"  force_bin_pt=on  bin_pt=0  block_type=cast
      settings: block_version=VER_STRING_GOES_HERE
  Reinterpret1 : xbsIndex_r4/Reinterpret  force_arith_type=on  arith_type=Unsigned  force_bin_pt=on  bin_pt=0  block_type=reinterpret
      settings: infoedit="Changes signal type without altering the binary representation.   You can changed the signal between signed and unsigned, and relocate the binary point.<br><br>Hardware notes: In hardware this block costs nothing.<br><br>Example:  Suppose the input is 6 bits wide, signed, with 2 fractional bits, and the output is forced to unsigned with 0 fractional bits.  Then an input of -2.0 (1110.00 in binary 2's complement) becomes an output of 56 (111000 in binary)."  block_version=8.2.02
  Reinterpret2 : xbsIndex_r4/Reinterpret  force_arith_type=on  arith_type=Unsigned  force_bin_pt=on  bin_pt=0  block_type=cast
      settings: block_version=VER_STRING_GOES_HERE
  Reinterpret3 : xbsIndex_r4/Reinterpret  force_arith_type=on  arith_type=Unsigned  force_bin_pt=on  bin_pt=0  block_type=cast
      settings: block_version=VER_STRING_GOES_HERE
  Reinterpret4 : xbsIndex_r4/Reinterpret  force_arith_type=on  arith_type=Unsigned  force_bin_pt=on  bin_pt=0  block_type=cast
      settings: block_version=VER_STRING_GOES_HERE
  Reinterpret5 : xbsIndex_r4/Reinterpret  force_arith_type=on  arith_type=Unsigned  force_bin_pt=on  bin_pt=0  block_type=reinterpret
      settings: block_version=8.2.02
  Reinterpret6 : xbsIndex_r4/Reinterpret  force_arith_type=on  arith_type=Unsigned  force_bin_pt=on  bin_pt=0  block_type=reinterpret
      settings: block_version=8.2.02
  Relational : xbsIndex_r4/Relational  mode=a=b  op_type=Bool  en=off  latency=1  dbl_ovrd=off  block_type=relational
  Relational1 : xbsIndex_r4/Relational  mode=a>b  op_type=Bool  en=off  latency=1  dbl_ovrd=off  block_type=relational
      settings: block_version=10.1
  Relational2 : xbsIndex_r4/Relational  mode=a=b  op_type=Bool  en=off  latency=1  dbl_ovrd=off  block_type=relational
  Relational3 : xbsIndex_r4/Relational  mode=a=b  op_type=Bool  en=off  latency=1  dbl_ovrd=off  block_type=relational
  ResetPicos : xbsIndex_r4/Gateway In  gui_display_data_type=Boolean  arith_type=Boolean  n_bits=1  bin_pt=0  preci_type=Single  exp_width=8  frac_width=24  rows=1  columns=1  quantization="Round  (unbiased: +/- Inf)"  overflow=Saturate  period=fpgaclk  UseAsADC=off  ADCChannel='1'  interface=None  automatic_assignment=on  address_offset=hex2dec('00')  intf_name=''  intf_description=''  default_value=0  timing_constraint=None  locs_specified=off  LOCs=RS232rx  io_standard={'LVCMOS33'}  inherit_from_input=off  hdl_port=on  dbl_ovrd=off  block_type=gatewayin
      settings: block_version=VER_STRING_GOES_HERE
  SCK : xbsIndex_r4/Gateway Out  inherit_from_input=off  hdl_port=on  rows=1  columns=1  UseAsDAC=off  DACChannel='1'  interface=None  automatic_assignment=on  address_offset=hex2dec('00')  intf_name=''  intf_description=''  timing_constraint=None  locs_specified=on  LOCs=SCK  io_standard={'LVCMOS33'}  block_type=gatewayout
      settings: xl_area=[0, 0, 0, 0, 0, 0, 0]  block_version=VER_STRING_GOES_HERE
  SCLK_BT : xbsIndex_r4/Gateway Out  inherit_from_input=off  hdl_port=on  rows=1  columns=1  UseAsDAC=off  DACChannel='1'  interface=None  automatic_assignment=on  address_offset=hex2dec('00')  intf_name=''  intf_description=''  timing_constraint=None  locs_specified=on  LOCs=SCLK_BT  io_standard={'LVCMOS33'}  block_type=gatewayout
      settings: block_version=VER_STRING_GOES_HERE
  SDOA : xbsIndex_r4/Gateway In  gui_display_data_type=Fixed-point  arith_type=Unsigned  n_bits=1  bin_pt=0  preci_type=Single  exp_width=8  frac_width=24  rows=1  columns=1  quantization="Round  (unbiased: +/- Inf)"  overflow=Saturate  period=fpgaclk  UseAsADC=off  ADCChannel='1'  interface=None  automatic_assignment=on  address_offset=hex2dec('00')  intf_name=''  intf_description=''  default_value=0  timing_constraint=None  locs_specified=on  LOCs=SDOA  io_standard={'LVCMOS33'}  inherit_from_input=off  hdl_port=on  dbl_ovrd=off  block_type=gatewayin
      settings: xl_area=[0, 0, 0, 0, 0, 0, 0]  block_version=VER_STRING_GOES_HERE
  SDOB : xbsIndex_r4/Gateway In  gui_display_data_type=Fixed-point  arith_type=Unsigned  n_bits=1  bin_pt=0  preci_type=Single  exp_width=8  frac_width=24  rows=1  columns=1  quantization="Round  (unbiased: +/- Inf)"  overflow=Saturate  period=fpgaclk  UseAsADC=off  ADCChannel='1'  interface=None  automatic_assignment=on  address_offset=hex2dec('00')  intf_name=''  intf_description=''  default_value=0  timing_constraint=None  locs_specified=on  LOCs=SDOB  io_standard={'LVCMOS33'}  inherit_from_input=off  hdl_port=on  dbl_ovrd=off  block_type=gatewayin
      settings: xl_area=[0, 0, 0, 0, 0, 0, 0]  block_version=VER_STRING_GOES_HERE
  SFS_BT : xbsIndex_r4/Gateway Out  inherit_from_input=off  hdl_port=on  rows=1  columns=1  UseAsDAC=off  DACChannel='1'  interface=None  automatic_assignment=on  address_offset=hex2dec('00')  intf_name=''  intf_description=''  timing_constraint=None  locs_specified=on  LOCs=SFS_BT  io_standard={'LVCMOS33'}  block_type=gatewayout
      settings: block_version=VER_STRING_GOES_HERE
  SRD_BT : xbsIndex_r4/Gateway Out  inherit_from_input=off  hdl_port=on  rows=1  columns=1  UseAsDAC=off  DACChannel='1'  interface=None  automatic_assignment=on  address_offset=hex2dec('00')  intf_name=''  intf_description=''  timing_constraint=None  locs_specified=on  LOCs=SRDBT  io_standard={'LVCMOS33'}  block_type=gatewayout
      settings: block_version=VER_STRING_GOES_HERE
  "SSBmodulator " : Subsystem
  STD_BT : xbsIndex_r4/Gateway In  gui_display_data_type=Fixed-point  arith_type=Unsigned  n_bits=1  bin_pt=0  preci_type=Single  exp_width=8  frac_width=24  rows=1  columns=1  quantization="Round  (unbiased: +/- Inf)"  overflow=Saturate  period=fpgaclk  UseAsADC=off  ADCChannel='1'  interface=None  automatic_assignment=on  address_offset=hex2dec('00')  intf_name=''  intf_description=''  default_value=0  timing_constraint=None  locs_specified=on  LOCs=STDBT  io_standard={'LVCMOS33'}  inherit_from_input=off  hdl_port=on  dbl_ovrd=off  block_type=gatewayin
      settings: block_version=VER_STRING_GOES_HERE
  Scope : Scope  NumInputPorts=2
      settings: YMin=0~7782.4  YMax=1~8601.6
  Scope1 : Scope
      settings: SaveName=ScopeData2
  Signed_Unsigned_offset : Subsystem
  Slice : xbsIndex_r4/Slice  nbits=1  boolean_output=off  mode=Lower Bit Location + Width  bit1=0  base1=MSB of Input  bit0=0  base0=LSB of Input  dbl_ovrd=off  block_type=slice
  Slice1 : xbsIndex_r4/Slice  nbits=3  boolean_output=off  mode=Lower Bit Location + Width  bit1=0  base1=MSB of Input  bit0=0  base0=LSB of Input  dbl_ovrd=off  block_type=slice
      settings: block_version=VER_STRING_GOES_HERE
  Slice10 : xbsIndex_r4/Slice  nbits=16  boolean_output=off  mode=Lower Bit Location + Width  bit1=0  base1=MSB of Input  bit0=0  base0=LSB of Input  dbl_ovrd=off  block_type=slice
      settings: block_version=VER_STRING_GOES_HERE
  Slice11 : xbsIndex_r4/Slice  nbits=3  boolean_output=off  mode=Lower Bit Location + Width  bit1=0  base1=MSB of Input  bit0=0  base0=LSB of Input  dbl_ovrd=off  block_type=slice
  Slice12 : xbsIndex_r4/Slice  nbits=1  boolean_output=off  mode=Lower Bit Location + Width  bit1=0  base1=MSB of Input  bit0=3  base0=LSB of Input  dbl_ovrd=off  block_type=slice
  Slice13 : xbsIndex_r4/Slice  nbits=2  boolean_output=off  mode=Lower Bit Location + Width  bit1=0  base1=MSB of Input  bit0=5  base0=LSB of Input  dbl_ovrd=off  block_type=slice
  Slice14 : xbsIndex_r4/Slice  nbits=1  boolean_output=off  mode=Lower Bit Location + Width  bit1=0  base1=MSB of Input  bit0=4  base0=LSB of Input  dbl_ovrd=off  block_type=slice
  Slice15 : xbsIndex_r4/Slice  nbits=1  boolean_output=off  mode=Lower Bit Location + Width  bit1=0  base1=MSB of Input  bit0=7  base0=LSB of Input  dbl_ovrd=off  block_type=slice
  Slice16 : xbsIndex_r4/Slice  nbits=1  boolean_output=off  mode=Lower Bit Location + Width  bit1=0  base1=MSB of Input  bit0=8  base0=LSB of Input  dbl_ovrd=off  block_type=slice
  Slice19 : xbsIndex_r4/Slice  nbits=8  boolean_output=off  mode=Upper Bit Location + Width  bit1=0  base1=MSB of Input  bit0=0  base0=LSB of Input  dbl_ovrd=off  block_type=slice
  Slice2 : xbsIndex_r4/Slice  nbits=1  boolean_output=off  mode=Lower Bit Location + Width  bit1=0  base1=MSB of Input  bit0=0  base0=LSB of Input  dbl_ovrd=off  block_type=slice
      settings: block_version=VER_STRING_GOES_HERE
  Slice3 : xbsIndex_r4/Slice  nbits=1  boolean_output=off  mode=Upper Bit Location + Width  bit1=0  base1=MSB of Input  bit0=0  base0=LSB of Input  dbl_ovrd=off  block_type=slice
      settings: block_version=VER_STRING_GOES_HERE
  Slice4 : xbsIndex_r4/Slice  nbits=1  boolean_output=off  mode=Upper Bit Location + Width  bit1=0  base1=MSB of Input  bit0=0  base0=LSB of Input  dbl_ovrd=off  block_type=slice
      settings: block_version=VER_STRING_GOES_HERE
  Slice5 : xbsIndex_r4/Slice  nbits=1  boolean_output=off  mode=Upper Bit Location + Width  bit1=0  base1=MSB of Input  bit0=0  base0=LSB of Input  dbl_ovrd=off  block_type=slice
      settings: block_version=VER_STRING_GOES_HERE
  Slice6 : xbsIndex_r4/Slice  nbits=1  boolean_output=off  mode=Lower Bit Location + Width  bit1=0  base1=MSB of Input  bit0=0  base0=LSB of Input  dbl_ovrd=off  block_type=slice
      settings: block_version=VER_STRING_GOES_HERE
  Slice7 : xbsIndex_r4/Slice  nbits=4  boolean_output=off  mode=Lower Bit Location + Width  bit1=0  base1=MSB of Input  bit0=20  base0=LSB of Input  dbl_ovrd=off  block_type=slice
      settings: block_version=VER_STRING_GOES_HERE
  Slice8 : xbsIndex_r4/Slice  nbits=1  boolean_output=off  mode=Lower Bit Location + Width  bit1=0  base1=MSB of Input  bit0=1  base0=LSB of Input  dbl_ovrd=off  block_type=slice
  Slice9 : xbsIndex_r4/Slice  nbits=3  boolean_output=off  mode=Lower Bit Location + Width  bit1=0  base1=MSB of Input  bit0=16  base0=LSB of Input  dbl_ovrd=off  block_type=slice
      settings: block_version=VER_STRING_GOES_HERE
  Stream_tdata : xbsIndex_r4/Gateway Out  inherit_from_input=off  hdl_port=on  rows=1  columns=1  UseAsDAC=off  DACChannel='1'  interface=None  automatic_assignment=on  address_offset=hex2dec('00')  intf_name=''  intf_description=''  timing_constraint=None  locs_specified=off  LOCs={}  io_standard={'LVCMOS33'}  block_type=gatewayout
      settings: block_version=VER_STRING_GOES_HERE
  Stream_tlast : xbsIndex_r4/Gateway Out  inherit_from_input=off  hdl_port=on  rows=1  columns=1  UseAsDAC=off  DACChannel='1'  interface=None  automatic_assignment=on  address_offset=hex2dec('00')  intf_name=''  intf_description=''  timing_constraint=None  locs_specified=off  LOCs={}  io_standard={'LVCMOS33'}  block_type=gatewayout
      settings: block_version=VER_STRING_GOES_HERE
  Stream_tready : xbsIndex_r4/Gateway In  gui_display_data_type=Boolean  arith_type=Boolean  n_bits=1  bin_pt=0  preci_type=Single  exp_width=8  frac_width=24  rows=1  columns=1  quantization="Round  (unbiased: +/- Inf)"  overflow=Saturate  period=fpgaclk  UseAsADC=off  ADCChannel='1'  interface=None  automatic_assignment=on  address_offset=hex2dec('00')  intf_name=''  intf_description=''  default_value=0  timing_constraint=None  locs_specified=off  LOCs=TouchOn  io_standard={'LVCMOS'}  inherit_from_input=off  hdl_port=on  dbl_ovrd=off  block_type=gatewayin
      settings: xl_area=[0, 0, 0, 0, 0, 0, 0]  block_version=VER_STRING_GOES_HERE
  Stream_tvalid : xbsIndex_r4/Gateway Out  inherit_from_input=off  hdl_port=on  rows=1  columns=1  UseAsDAC=off  DACChannel='1'  interface=None  automatic_assignment=on  address_offset=hex2dec('00')  intf_name=''  intf_description=''  timing_constraint=None  locs_specified=off  LOCs={}  io_standard={'LVCMOS33'}  block_type=gatewayout
      settings: block_version=VER_STRING_GOES_HERE
  Strobe : xbsIndex_r4/Gateway Out  inherit_from_input=off  hdl_port=on  rows=1  columns=1  UseAsDAC=off  DACChannel='1'  interface=None  automatic_assignment=on  address_offset=hex2dec('00')  intf_name=''  intf_description=''  timing_constraint=None  locs_specified=on  LOCs=Strobe  io_standard={'LVCMOS33'}  block_type=gatewayout
      settings: block_version=VER_STRING_GOES_HERE
  StrobeTones : xbsIndex_r4/Gateway Out  inherit_from_input=off  hdl_port=on  rows=1  columns=1  UseAsDAC=off  DACChannel='1'  interface=None  automatic_assignment=on  address_offset=hex2dec('00')  intf_name=''  intf_description=''  timing_constraint=None  locs_specified=off  LOCs={}  io_standard={'LVCMOS33'}  block_type=gatewayout
      settings: block_version=VER_STRING_GOES_HERE
  Subsystem1 : Subsystem
  Subsystem2 : Subsystem
  Subsystem4 : Subsystem
  TX_Low : xbsIndex_r4/Gateway Out  inherit_from_input=off  hdl_port=on  rows=1  columns=1  UseAsDAC=off  DACChannel='1'  interface=None  automatic_assignment=on  address_offset=hex2dec('00')  intf_name=''  intf_description=''  timing_constraint=None  locs_specified=on  LOCs=TX_LOW  io_standard={'LVCMOS33'}  block_type=gatewayout
      settings: block_version=VER_STRING_GOES_HERE
  ToneDetect : Subsystem
  Touch{1..4} (4 alike) : xbsIndex_r4/Register  init=0  rst=off  en=off  dbl_ovrd=off  block_type=register
      settings: xl_area=[0, 0, 0, 0, 0, 0, 0]  block_version=VER_STRING_GOES_HERE
  TouchDown : xbsIndex_r4/Gateway In  gui_display_data_type=Fixed-point  arith_type=Unsigned  n_bits=1  bin_pt=0  preci_type=Single  exp_width=8  frac_width=24  rows=1  columns=1  quantization="Round  (unbiased: +/- Inf)"  overflow=Saturate  period=fpgaclk  UseAsADC=off  ADCChannel='1'  interface=None  automatic_assignment=on  address_offset=hex2dec('00')  intf_name=''  intf_description=''  default_value=0  timing_constraint=None  locs_specified=on  LOCs=TouchDown  io_standard={'LVCMOS'}  inherit_from_input=off  hdl_port=on  dbl_ovrd=off  block_type=gatewayin
      settings: xl_area=[0, 0, 0, 0, 0, 0, 0]  block_version=VER_STRING_GOES_HERE
  TouchOn : xbsIndex_r4/Gateway In  gui_display_data_type=Fixed-point  arith_type=Unsigned  n_bits=1  bin_pt=0  preci_type=Single  exp_width=8  frac_width=24  rows=1  columns=1  quantization="Round  (unbiased: +/- Inf)"  overflow=Saturate  period=fpgaclk  UseAsADC=off  ADCChannel='1'  interface=None  automatic_assignment=on  address_offset=hex2dec('00')  intf_name=''  intf_description=''  default_value=0  timing_constraint=None  locs_specified=on  LOCs=TouchOn  io_standard={'LVCMOS'}  inherit_from_input=off  hdl_port=on  dbl_ovrd=off  block_type=gatewayin
      settings: xl_area=[0, 0, 0, 0, 0, 0, 0]  block_version=VER_STRING_GOES_HERE
  TouchSelect : xbsIndex_r4/Gateway In  gui_display_data_type=Fixed-point  arith_type=Unsigned  n_bits=1  bin_pt=0  preci_type=Single  exp_width=8  frac_width=24  rows=1  columns=1  quantization="Round  (unbiased: +/- Inf)"  overflow=Saturate  period=fpgaclk  UseAsADC=off  ADCChannel='1'  interface=None  automatic_assignment=on  address_offset=hex2dec('00')  intf_name=''  intf_description=''  default_value=0  timing_constraint=None  locs_specified=on  LOCs=TouchSelect  io_standard={'LVCMOS'}  inherit_from_input=off  hdl_port=on  dbl_ovrd=off  block_type=gatewayin
      settings: xl_area=[0, 0, 0, 0, 0, 0, 0]  block_version=VER_STRING_GOES_HERE
  TouchUp : xbsIndex_r4/Gateway In  gui_display_data_type=Fixed-point  arith_type=Unsigned  n_bits=1  bin_pt=0  preci_type=Single  exp_width=8  frac_width=24  rows=1  columns=1  quantization="Round  (unbiased: +/- Inf)"  overflow=Saturate  period=fpgaclk  UseAsADC=off  ADCChannel='1'  interface=None  automatic_assignment=on  address_offset=hex2dec('00')  intf_name=''  intf_description=''  default_value=0  timing_constraint=None  locs_specified=on  LOCs=TouchUp  io_standard={'LVCMOS33'}  inherit_from_input=off  hdl_port=on  dbl_ovrd=off  block_type=gatewayin
      settings: xl_area=[0, 0, 0, 0, 0, 0, 0]  block_version=VER_STRING_GOES_HERE
  User_Interface : Subsystem
  Values2Recover : xbsIndex_r4/Gateway In  gui_display_data_type=Fixed-point  arith_type=Unsigned  n_bits=32  bin_pt=0  preci_type=Single  exp_width=8  frac_width=24  rows=1  columns=1  quantization="Round  (unbiased: +/- Inf)"  overflow=Saturate  period=fpgaclk  UseAsADC=off  ADCChannel='1'  interface=AXI4-Lite  automatic_assignment=on  address_offset=hex2dec('00')  intf_name=''  intf_description=''  default_value=0  timing_constraint=None  locs_specified=off  LOCs=RS232rx  io_standard={'LVCMOS33'}  inherit_from_input=off  hdl_port=on  dbl_ovrd=off  block_type=gatewayin
      settings: block_version=VER_STRING_GOES_HERE
  tag scope: ADCSignalLevel=global, ADCStrobe=global, ADCchA=global, ADCchB=global, ADCpeak=global, ARM_ADCselect=global, ARM_Beaconselect=global, ARM_ResetPicos=global, ARM_Voice_TextMode=global, Address=global, AudioAmp=global, AudioOut=global, AudioVolume=global, BTAudio=global, DataFromARM=global, Demodpeak=global, Dim=global, FilterredSignal=global, Instruction=global, KPdata2Archive=global, KPdata2Archive_W=global, MessageInjectionSelect=global, NoBTsignal=global, RateLoranTrips=global, RdyforUserTxData=global, RstPicos=global, Square128kHz=global, Square8kHz=global, Strobe=global, TX_High=global, TXtone=global, ToSpeaker=global, ToneDetectOff=global, ValidFromARM=global
  wires:
  ADCRead/1(SCK) -> SCK/1
  SDOA/1 -> ADCRead/1(SDOA)
  ADCRead/2(CONV) -> CONV/1
  PWMAudio/1 -> Scope/1
  DAC (XAPP154)1/1(DAC_Out) -> PWMAudio/1
  ADCtrigger/1(Trig512) -> Convert1/1
  Convert1/1 -> ADCRead/3(Trig), Counter3/1
  ADCRead/4(Data_Ready) -> Delay1/1
  Reinterpret/1 -> Slice19/1, Signed_Unsigned_offset/1(In1)
  Subsystem2/2(CleanedUp) -> Reinterpret1/1, DemodulationSSB1/1(SignalIn)
  DemodulationSSB1/1(DemodSignal) -> [FilterredSignal], DSProcessor1/1(FilterredSignal)
  User_Interface/3(Addressb) -> ArchiveRam/4, [Address]
  User_Interface/4(Instruction) -> [Instruction]
  Counter/1 -> ArchiveRam/1
  ArchiveRam/2 -> User_Interface/1(ArchivedData)
  Mux2/1 -> ArchiveRam/2
  Monostable/1 -> Counter/1
  User_Interface/7(Enable Archive) -> Monostable/1, Logical/1
  User_Interface/8(Select_source) -> Slice6/1
  DSProcessor1/4(Data2Archive) -> LevelMonitor1/1(In1), Mux2/3
  DemodulationSSB1/2(DemodSqStrobe) -> Convert2/1, [Strobe], DSProcessor1/4(Strobe), Strobe/1
  Mux3/1 -> Counter/2, Logical/2
  Logical/1 -> Convert5/1
  User_Interface/5(PicoCmd) -> DSProcessor1/2(Cmd)
  DSProcessor1/2(Amp) -> [AudioAmp], "SSBmodulator "/1(AudioAmp)
  "SSBmodulator "/1(HinA) -> ClassD_HinA/1
  "SSBmodulator "/2(HinB) -> ClassD_HinB/1
  User_Interface/6(NewCmd) -> DSProcessor1/3(NewCmd)
  Constant4/1 -> ArchiveRam/6
  Constant5/1 -> ArchiveRam/5
  Monostable1/1 -> Mux3/3, LevelMonitor1/2(En), Counter1/1
  Convert2/1 -> Monostable1/1, [Square8kHz]
  DSProcessor1/3(CmdToUser) -> User_Interface/2(CmdFromDSP)
  DSProcessor1/6(NewCmdToUser) -> User_Interface/3(NewCmdFromDSP)
  User_Interface/11(ADCgain) -> Concat6/1, Concat4/3, ADC_Gain/1  "ADCGain"
  Relational1/1 -> LCDContrast/1
  [Counter6kHz] -> Relational1/2
  [LCDcontrast] -> Relational1/1
  User_Interface/12(CAL) -> ADC_CAL/1
  SDOB/1 -> ADCRead/2(SDOB)
  ADCRead/3(ADC_Data_A) -> Bit_Corrector/1(In1)
  ADCRead/5(ADC_Data_B) -> Bit_Corrector1/1(In1)
  Delay1/1 -> [ADCStrobe], Mux3/2, DemodulationSSB1/2(Trig), Subsystem2/2(Strbe), LoranPulsedetect/2(Strobe), LevelMonitor/2(En)
  KeyPadinterface/4(LCDctrl) -> Slice1/1
  LCDdata/1 -> Display/1
  Slice1/1 -> LCDctrl/1
  KeyPadinterface/3(LCDdata) -> LCDdata/1
  KeyPadinterface/2(Data2Archive_W) -> [KPdata2Archive_W]
  KeyPadinterface/1(Data2Archive) -> [KPdata2Archive]
  Slice6/1 -> Mux2/1, Mux3/1
  Convert5/1 -> ArchiveRam/3
  Mux1/1 -> LevelMonitor/1(In1), LoranPulsedetect/1(Signal), Subsystem2/1(Signal)
  KeyPadinterface/5(LatchOn) -> Slice2/1
  TouchUp/1 -> Touch1/1
  TouchDown/1 -> Touch2/1
  TouchSelect/1 -> Touch3/1
  [BTAudio] -> DSProcessor1/5(BTauidioIN)
  [ADCselect] -> Mux1/1
  "SSBmodulator "/3(LinA) -> ClassD_LinA/1
  "SSBmodulator "/4(LinB) -> ClassD_LinB/1
  Constant1/1 -> Concat1/1
  CoutA1/1 -> Concat1/3
  Concat1/1 -> KeyPadinterface/1(TouchSignal)
  Bit_Corrector/1(Out1) -> Mux1/2, Reinterpret6/1
  Bit_Corrector1/1(Out1) -> Mux1/3, Reinterpret5/1
  Reinterpret1/1 -> Mux2/2
  LevelMonitor/1(SignalLevel) -> Concat6/2, [ADCSignalLevel], User_Interface/4(ADCSignalLevel)
  DSProcessor1/7(TX_Phase) -> "SSBmodulator "/4(TXphase)
  PTT/1 -> CoutA1/1
  LoranPulsedetect/1(Trig) -> Subsystem2/3(LoranPulseTrig)
  [TX_High] -> Inverter1/1
  [LoranBlankselect] -> Logical1/1
  Inverter1/1 -> Logical1/2
  Logical1/1 -> Subsystem2/4(EnableGating)
  DSProcessor1/5(PhaseIncrement 8bits) -> "SSBmodulator "/5(PhaseIncrement)
  DSProcessor1/8(NewValue) -> "SSBmodulator "/6(NewPhaseValue)
  Counter1/1 -> Slice4/1
  Slice4/1 -> Convert3/1
  Monostable3/1 -> Counter2/1, NoTrips/2
  Counter2/1 -> NoTrips/1
  NoTrips/1 -> [RateLoranTrips]
  [LoranTrig] -> Counter2/2
  Convert3/1 -> Monostable3/1
  [NoBTsignal] -> Inverter2/1
  Subsystem4/3(SFS) -> Subsystem1/3(SFS), SFS_BT/1
  Subsystem4/2(128kHz) -> Subsystem1/2(128kHz), Monostable2/1, SCLK_BT/1
  Subsystem4/1(PCMout) -> SRD_BT/1
  SRD_BT/1 -> STD_BT/1
  ConstantDetect/1(IsConstant) -> Logical4/2, Inverter5/1, [NoBTsignal]
  STD_BT/1 -> ConstantDetect/1(Signal), Subsystem1/1(PCMin)
  Counter3/1 -> Slice3/1
  Slice3/1 -> [Square128kHz]
  Slice5/1 -> Convert4/1
  Convert4/1 -> Monostable4/1
  Monostable2/1 -> Counter4/1
  Monostable4/1 -> Counter5/1, ConstantDetect/2(Strobe)
  Counter4/1 -> Slice5/1
  Constant2/1 -> Concat2/1
  Touch1/1 -> Concat2/2
  Touch2/1 -> Concat2/3
  Touch3/1 -> Concat2/4
  Concat2/1 -> KeyPadinterface/2(TouchSignal1)
  TouchOn/1 -> Touch4/1
  Touch4/1 -> Concat2/5
  [Attenuator] -> Slice8/1, Slice/1
  Slice2/1 -> KeepOn/1
  LevelMonitor/2(PkSignal) -> Concat6/3, [ADCpeak]
  [ResetPeak] -> LevelMonitor/3(RstPeak)
  LevelMonitor1/1(PkSignal) -> [Demodpeak]
  [ResetPeak] -> LevelMonitor1/3(RstPeak)
  User_Interface/9(TX_high) -> Inverter4/1, [TX_High], Delay16ms/1(In1)
  [TXFreq] -> "SSBmodulator "/2(CarrierFreq)
  User_Interface/10(TXtone) -> [TXtone]
  Signed_Unsigned_offset/1(Out1) -> DAC (XAPP154)1/1(DAC_In), Scope/2
  Inverter4/1 -> Convert/1, TX_Low/1
  ADCtrigger/2(Dim) -> [Dim]
  Logical2/1 -> LEDR/1
  Logical3/1 -> LEDG/1
  [Dim] -> Logical3/2, Logical2/2, Logical4/1
  Convert/1 -> Logical2/1
  Convert10/1 -> Logical3/1, DAC (XAPP154)1/2(Disable_Audio)
  Delay16ms/1(Out1) -> "SSBmodulator "/3(TX_enable)
  ADCtrigger/3(Clk1MHz) -> PSUclk/1
  Slice8/1 -> Match_Z/1
  Counter5/1 -> ROM/1
  Subsystem1/1(AudioOut) -> [BTAudio]
  [BTAudioOut] -> Subsystem4/1(AudioIn)
  DSProcessor1/1(AudioOut) -> [AudioOut], Reinterpret/1
  AudioVolume/1 -> [AudioVolume]
  [WriteUserTxData] -> Delay3/1
  [ARMdataAck] -> Convert8/1
  Inverter/1 -> PS2PL_tready/1
  PL2PS_tready/1 -> [RdyforUserTxData]
  Convert7/1 -> [ValidFromARM]
  Logical7/1 -> Counter6/2, Delay/1
  Logical5/1 -> Stream_tlast/1
  Constant3/1 -> Relational3/1  "LF"
  Relational3/1 -> Logical6/1
  Logical6/1 -> PL2PS_tlast/1
  [UserTxData] -> Relational3/2, PL2PS_tdata/1
  Delay3/1 -> Logical6/2, Delay4/1
  Delay4/1 -> PL2PS_tvalid/1
  Counter6/1 -> DataCounter/1, Relational/1
  Slice10/1 -> Relational2/1, Relational/2
  Relational/1 -> Logical9/2, Logical5/2
  Delay/1 -> Logical5/1, Stream_tvalid/1
  [FilterredSignal] -> Reinterpret3/1
  [Strobe] -> Monostable5/1
  Concat4/1 -> Mux/2
  Values2Recover/1 -> Slice7/1, Slice10/1, Slice9/1
  Slice9/1 -> Mux4/1, Mux/1
  Mux4/1 -> Logical7/1
  Monostable5/1 -> Convert9/1
  Constant6/1 -> Relational2/2
  Stream_tready/1 -> Logical8/1
  Latch/1 -> Inverter7/1, Logical8/2
  Logical8/1 -> Logical7/2
  Relational2/1 -> Inverter3/1, Logical9/1
  Logical9/1 -> Latch/2
  Inverter3/1 -> Monostable7/1
  Monostable7/1 -> Latch/1
  [AudioOut] -> Reinterpret4/1
  [BTAudio] -> Reinterpret2/1
  Concat5/1 -> Mux/3
  [StartTones] -> Mux/4
  [StopTones] -> Mux/5
  Mux/1 -> Stream_tdata/1
  [StrobeTones] -> StrobeTones/1, Mux4/7, Mux4/6, Mux4/5, Mux4/4
  Reinterpret3/1 -> Concat4/4
  Reinterpret2/1 -> Concat5/1
  Reinterpret4/1 -> Concat5/2
  Convert9/1 -> Mux4/3, Mux4/2, Mux4/9
  PS2PL_tdata/1 -> FIFO/1
  FIFO/4 -> Inverter/1
  Inverter6/1 -> Convert7/1
  FIFO/2 -> Inverter6/1
  FIFO/1 -> [DataFromARM]
  PS2PL_tvalid/1 -> FIFO/2
  Convert8/1 -> FIFO/3
  Inverter7/1 -> Counter6/1
  Logical4/1 -> LEDB/1
  [IQStartTones] -> Mux/6
  [IQStopTones] -> Mux/7
  [SpeakerOn] -> Inverter8/1
  Inverter8/1 -> Convert10/1
  Concat6/1 -> ADCgain_ave_peak/1
  [ADCStrobe] -> Mux4/8
  [ADCchA] -> Concat7/1
  [ADCchB] -> Concat7/2
  Concat7/1 -> Mux/8
  SCK/1 -> Scope1/1
  Reinterpret6/1 -> [ADCchA]
  Reinterpret5/1 -> [ADCchB]
  [AGCvalue] -> Concat4/2
  Constant7/1 -> Concat4/1
  Slice7/1 -> [MessageInjectionSelect]
  Slice19/1 -> [ToSpeaker]
  [TX_High] -> Mux5/1
  [ToSpeaker] -> Mux5/2
  [AudioAmp] -> Mux5/3
  Mux5/1 -> Concat8/1
  [AfterFilter] -> Concat8/3
  [AfterAGC] -> Concat8/4
  Concat8/1 -> Mux/9  "AudioLevelMonitor"
  [ArchiveMSB] -> Concat8/2
  N3Zconfig/1 -> Slice11/1, Slice16/1, Slice15/1, Slice13/1, Slice14/1, Slice12/1
  Slice11/1 -> Concat1/2
  Slice12/1 -> [ARM_ADCselect]
  Slice13/1 -> [ARM_Beaconselect]
  Slice14/1 -> [ARM_Voice_TextMode]
  Slice15/1 -> [ToneDetectOff]
  Slice16/1 -> [ARM_ResetPicos]
  ResetPicos/1 -> Logical10/1
  Logical10/1 -> [RstPicos]
  [ARM_ResetPicos] -> Convert6/1
  Convert6/1 -> Logical10/2
